simulink model "sampling_theroem"  (R2024a)
settings: Solver=VariableStepAuto  StartTime=0.0  StopTime=10  RelTol=1e-3
libraries: dspfdesign x1

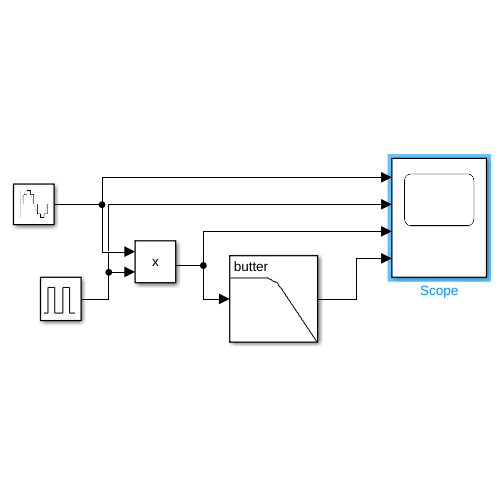
[thumbnail: Simulink's stored preview of the top-level diagram]
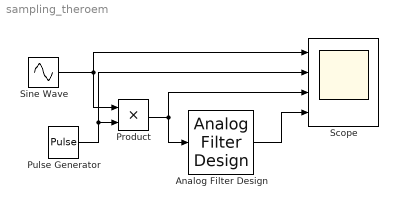
== system sampling_theroem ==
  Analog Filter Design : dspfdesign/Analog Filter Design  method=Butterworth  filttype=Lowpass  N=3  Wlo=1  Whi=80  Rp=2  Rs=40
  Product : Product
  Pulse Generator : DiscretePulseGenerator  PulseType=Time based  Period=0.025  PulseWidth=5
  Scope : Scope  NumInputPorts=4
  Sine Wave : Sin  Amplitude=2  Frequency=1.5  SampleTime=0.001
  wires:
  Product/1 -> Scope/3, Analog Filter Design/1
  Pulse Generator/1 -> Scope/2, Product/2
  Sine Wave/1 -> Product/1, Scope/1
  Analog Filter Design/1 -> Scope/4
